simulink model "untitled1"  (R2018a)
settings: Solver=VariableStepAuto  StartTime=0.0  StopTime=200  RelTol=1e-3
InitFcn:
  | init
undefined symbols (not defined in the file or in its folder): globtonextframe
libraries: simulink x2
settings Model: Creator=kyniu  LastModifiedBy=kyniu

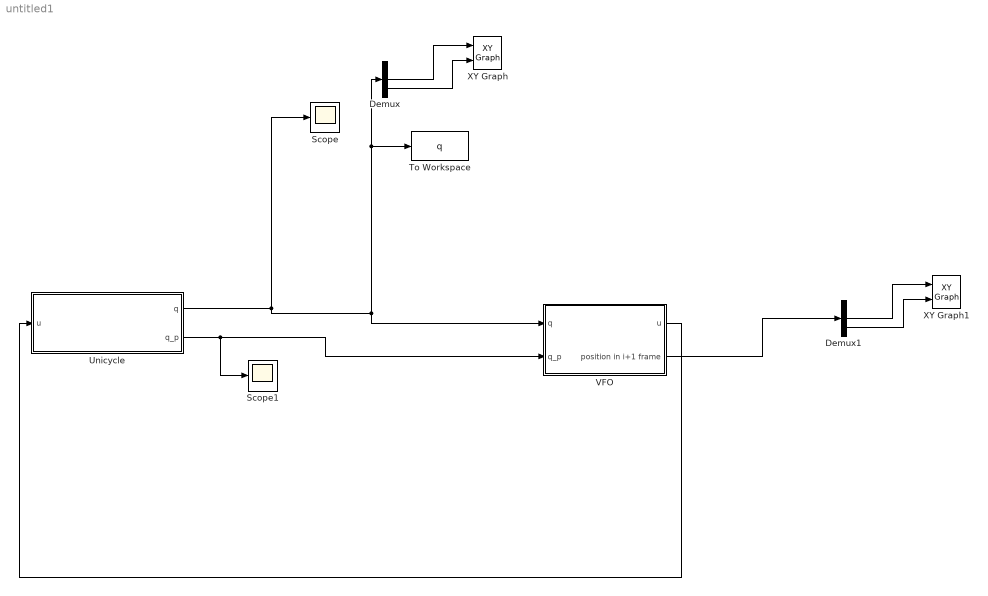
== system untitled1 ==
  Demux : Demux  Outputs=3
  Demux1 : Demux  Outputs=3
  Scope : Scope
  Scope1 : Scope
  To Workspace : ToWorkspace  VariableName=q  SaveFormat=Timeseries  SampleTime=-1
  Unicycle : Subsystem
  VFO : Subsystem
  XY Graph : simulink/Sinks/XY Graph  xmin=0  xmax=100  ymin=0  ymax=100  st=-1
  XY Graph1 : simulink/Sinks/XY Graph  xmin=0  xmax=100  ymin=0  ymax=100  st=-1
  wires:
  VFO/1("u ") -> Unicycle/1(u)
  Unicycle/2(q_p) -> Scope1/1, VFO/2(q_p)
  Unicycle/1(q) -> VFO/1(q), Demux/1, To Workspace/1, Scope/1
  Demux/2 -> XY Graph/1
  Demux/3 -> XY Graph/2
  Demux1/2 -> XY Graph1/1
  Demux1/3 -> XY Graph1/2
  VFO/2(position in i+1 frame) -> Demux1/1

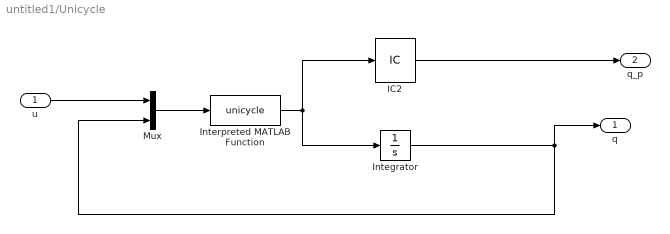
== system untitled1/Unicycle ==
  u : Inport
  IC2 : InitialCondition  Value=[0;0;0]
  Integrator : Integrator  InitialCondition=[0;0;0]
  Interpreted MATLAB Function : MATLABFcn  MATLABFcn=unicycle
  Mux : Mux  Inputs=2
  q : Outport
  q_p : Outport  Port=2
  wires:
  Integrator/1 -> q/1, Mux/2
  IC2/1 -> q_p/1
  Mux/1 -> Interpreted MATLAB Function/1
  Interpreted MATLAB Function/1 -> Integrator/1, IC2/1
  u/1 -> Mux/1

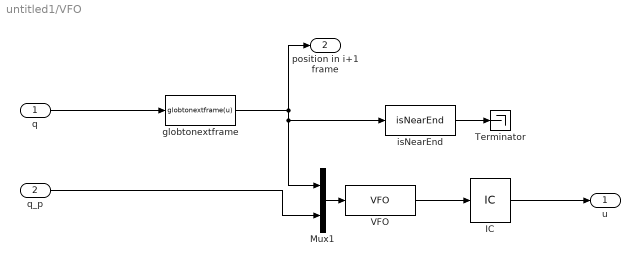
== system untitled1/VFO ==
  q : Inport
  q_p : Inport  Port=2
  IC : InitialCondition  Value=[0;0]
  Mux1 : Mux  Inputs=2
  Terminator : Terminator
  VFO : MATLABFcn  MATLABFcn=VFO
  globtonextframe : MATLABFcn  MATLABFcn=globtonextframe(u)
  "isNearEnd " : MATLABFcn  MATLABFcn=isNearEnd
  "u " : Outport
  position in i+1 frame : Outport  Port=2
  wires:
  Mux1/1 -> VFO/1
  VFO/1 -> IC/1
  IC/1 -> "u "/1
  q_p/1 -> Mux1/2
  globtonextframe/1 -> position in i+1 frame/1, "isNearEnd "/1, Mux1/1
  q/1 -> globtonextframe/1
  "isNearEnd "/1 -> Terminator/1
